simulink model "buck_boost_converter"  (R2024a)
settings: Solver=VariableStepAuto  StartTime=0.0  StopTime=.15  RelTol=1e-3
libraries: spsSeriesRLCBranchLib x3, spsCurrentMeasurementLib x2, spsVoltageMeasurementLib x2, spsDCVoltageSourceLib x1, spsDiodeLib x1, spsGroundLib x1, spsMeanLib x1, spsMosfetLib x1, spsPWMGeneratorDCDCLib x1, sps_lib x1, spspowerguiLib x1
settings Model: Creator=Jagan mohan  LastModifiedBy=Jagan mohan

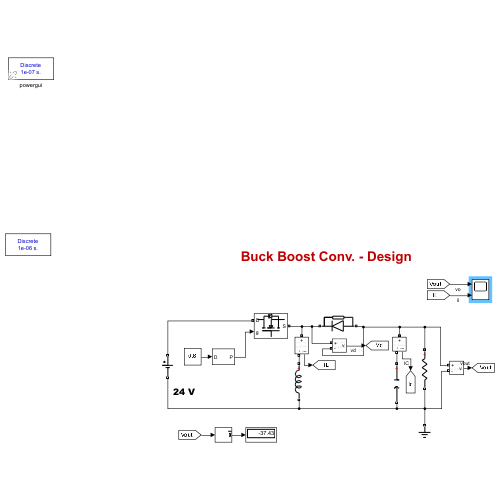
[thumbnail: Simulink's stored preview of the top-level diagram]
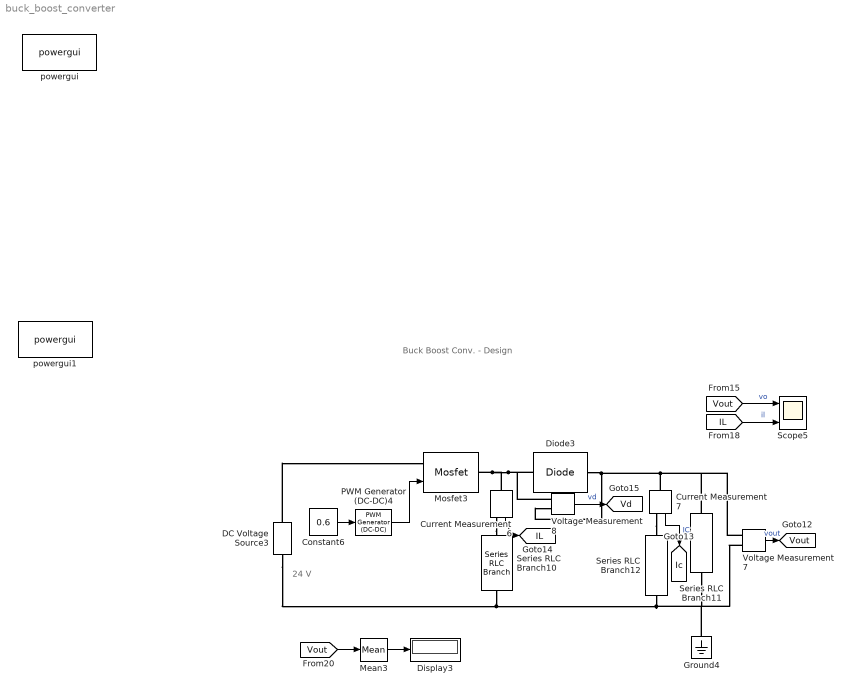
== system buck_boost_converter ==
  note: 24 V
  note: Buck Boost Conv. - Design
  Constant6 : Constant  Value=0.6
  Current Measurement6 : spsCurrentMeasurementLib/Current Measurement  PhasorSimulation=off  OutputType=Complex  PSBequivalent=0
  Current Measurement7 : spsCurrentMeasurementLib/Current Measurement  PhasorSimulation=off  OutputType=Complex  PSBequivalent=0
  DC Voltage Source3 : spsDCVoltageSourceLib/DC Voltage Source  Amplitude=24  Measurements=None
  Diode3 : spsDiodeLib/Diode  Ron=1e-7  Lon=0  Vf=0  IC=0  UseSnubber=0  Rs=1e6  Cs=1e6  Measurements=off
  Display3 : Display
  Ground4 : spsGroundLib/Ground  LConnTagsString=a
  Mean3 : spsMeanLib/Mean  Freq=10000  Vinit=0  Ts=0
  Mosfet3 : spsMosfetLib/Mosfet  Ron=1e-7  Lon=0  Rd=1e-10  Vfd=0  IC=0  Rs=inf  Cs=0  Measurements=off
  PWM Generator (DC-DC)4 : spsPWMGeneratorDCDCLib/PWM Generator (DC-DC)  Fsw=10000  Ts=1e-6
  Scope5 : Scope  NumInputPorts=2
  Series RLC Branch10 : spsSeriesRLCBranchLib/Series RLC Branch  LConnTagsString=__new0  RConnTagsString=__new0  BranchType=L  Resistance=0.000001  Inductance=0.0144  SetiL0=off  InitialCurrent=0  Capacitance=1e-6  Setx0=off  InitialVoltage=0  Measurements=None
  Series RLC Branch11 : spsSeriesRLCBranchLib/Series RLC Branch  LConnTagsString=__new0  RConnTagsString=__new0  BranchType=R  Resistance=18  Inductance=1e-3  SetiL0=off  InitialCurrent=0  Capacitance=1000e-6  Setx0=on  InitialVoltage=800  Measurements=None
  Series RLC Branch12 : spsSeriesRLCBranchLib/Series RLC Branch  LConnTagsString=__new0  RConnTagsString=__new0  BranchType=C  Resistance=6  Inductance=1e-3  SetiL0=off  InitialCurrent=0  Capacitance=66.67e-6  Setx0=off  InitialVoltage=800  Measurements=None
  Voltage Measurement7 : spsVoltageMeasurementLib/Voltage Measurement  PhasorSimulation=off  OutputType=Complex  PSBequivalent=0
  Voltage Measurement8 : spsVoltageMeasurementLib/Voltage Measurement  PhasorSimulation=off  OutputType=Complex  PSBequivalent=0
  powergui : sps_lib/powergui  Priority=1  SimulationMode=Discrete  SampleTime=10e-8  frequency=60  Iterations=50  frequencyindice=0  Pbase=100e6  ErrMax=1e-4  UnitsV=kV  UnitsW=MW  buscounter=0  FunctionMessages=off  echomessages=off  EnableUseOfTLC=off  CurrentSourceSwitches=off  DisableSnubberDevices=off  DisableRonSwitches=off  DisableVfSwitches=off  DisplayEquations=off  AutomaticDiscreteSolvers=off  SolverType=Tustin/Backward Euler (TBE)  Interpol=off  ExternalGateDelay=off  methode=off  Ts=100  x0status=blocks  SPID=on  SwTol=0  HookPort=off  NonlinearTolerance=1e-4  nMaxIteration=100  ContinueOnMaxIteration=off  RestoreLinks=warning  ResistiveCurrentMeasurement=off  Frange=[0:2:500]  Ylog=off  Xlog=on  ShowGrid=off  save=off  variable=ZData  structure=0  ZoomFFT=off  StartTime=0.0  cycles=1  DisplayStyle=1  fundamental=60  FreqAxis=off  MaxFrequency=1000  frequencyindicesteady=1  RmsSteady=1  display=off
  powergui1 : spspowerguiLib/powergui  Priority=1  SimulationMode=Discrete  SampleTime=1e-6  frequency=60  Iterations=50  frequencyindice=60  Pbase=100e6  ErrMax=1e-4  UnitsV=kV  UnitsW=MW  buscounter=0  FunctionMessages=off  echomessages=off  EnableUseOfTLC=off  CurrentSourceSwitches=off  DisableSnubberDevices=off  DisableRonSwitches=off  DisableVfSwitches=off  DisplayEquations=off  AutomaticDiscreteSolvers=off  SolverType=Tustin/Backward Euler (TBE)  Interpol=off  ExternalGateDelay=off  methode=off  Ts=100  x0status=blocks  SPID=on  SwTol=0  HookPort=off  NonlinearTolerance=1e-4  nMaxIteration=100  ContinueOnMaxIteration=off  RestoreLinks=warning  ResistiveCurrentMeasurement=off  Frange=[0:2:500]  Ylog=off  Xlog=on  ShowGrid=off  save=off  variable=ZData  structure=0  ZoomFFT=off  StartTime=0.0  cycles=1  DisplayStyle=1  fundamental=60  FreqAxis=off  MaxFrequency=1000  frequencyindicesteady=1  RmsSteady=1  display=off
  tag scope: IL=global, Ic=global, Vd=global, Vout=global
  wires:
  [Vout] -> Mean3/1
  [Vout] -> Scope5/1  "vo"
  Current Measurement6/1 -> [IL]
  [IL] -> Scope5/2  "il"
  Mean3/1 -> Display3/1
  Voltage Measurement8/1 -> [Vd]  "vd"
  Constant6/1 -> PWM Generator (DC-DC)4/1
  Voltage Measurement7/1 -> [Vout]  "vout"
  Current Measurement7/1 -> [Ic]  "IC"
  PWM Generator (DC-DC)4/1 -> Mosfet3/1
  connections:
  Current Measurement7/LConn1 -- Diode3/LConn1 -- Voltage Measurement8/LConn2 -- Series RLC Branch11/LConn1 -- Voltage Measurement7/LConn1
  Series RLC Branch10/RConn1 -- DC Voltage Source3/LConn1 -- Series RLC Branch11/RConn1 -- Voltage Measurement7/LConn2 -- Ground4/LConn1 -- Series RLC Branch12/RConn1
  Mosfet3/RConn1 -- Current Measurement6/LConn1 -- Diode3/RConn1 -- Voltage Measurement8/LConn1
  Current Measurement6/RConn1 -- Series RLC Branch10/LConn1
  Current Measurement7/RConn1 -- Series RLC Branch12/LConn1
  DC Voltage Source3/RConn1 -- Mosfet3/LConn1
